simulink model "ARXTest"  (R2019a)
settings: Solver=FixedStepAuto  StartTime=0.0  StopTime=5  FixedStep=Ts  RelTol=1e-3
model workspace (MAT data in the model file):
  Ts = 0.1
settings Model: Creator=Administrator  LastModifiedBy=Administrator

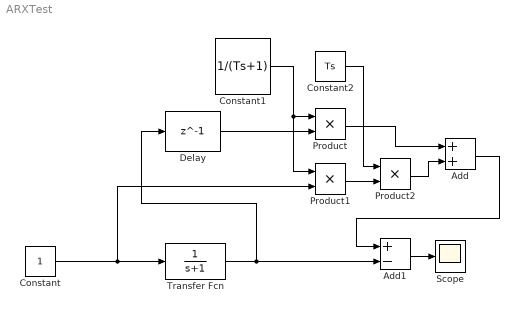
== system ARXTest ==
  Add : Sum
  Add1 : Sum  Inputs=+-
  Constant : Constant
  Constant1 : Constant  Value=1/(Ts+1)
  Constant2 : Constant  Value=Ts
  Delay : Delay  DelayLength=1  InitialCondition=0  UseCircularBuffer=on
  Product : Product
  Product1 : Product
  Product2 : Product
  Scope : Scope
  Transfer Fcn : TransferFcn  Denominator=[1 1]
  wires:
  Constant/1 -> Product1/2, Transfer Fcn/1
  Transfer Fcn/1 -> Add1/2, Delay/1
  Constant1/1 -> Product1/1, Product/1
  Delay/1 -> Product/2
  Product/1 -> Add/1
  Product1/1 -> Product2/2
  Constant2/1 -> Product2/1
  Product2/1 -> Add/2
  Add/1 -> Add1/1
  Add1/1 -> Scope/1
